simulink model "NavFilterTestHarness24"  (R2024b)
settings: Solver=FixedStepDiscrete  StartTime=startTime  StopTime=endTime  FixedStep=0.001  RelTol=1e-3  EnableMultiTasking=on
undefined symbols (not defined in the file): accel, ADSframe, ADStime, alignTime, angRate, ATTframe, CourseDeg, EAS2TAS, GndSpd, GPSframe, GPStime, Hgt, IMUframe, IMUtime, LatDeg, LngDeg, MagBiasX, MagBiasY, MagBiasZ, MAGframe, MAGtime, MagX, MagY, MagZ, msecHgtDelay, msecMagDelay, msecPosDelay, msecTasDelay, msecVelDelay, Pitch, Roll, Veas, VelD, Yaw
libraries: simulink x9, simulink_need_slupdate x2
(part 3 of 5)

== matlab function NavFilterTestHarness24/WatchDog/wrapAnglePi ==
  data: angleOut output; angleIn input
function angleOut   = wrapAnglePi(angleIn)
%#codegen

if abs(angleIn) <= pi
    angleOut = angleIn;
elseif  angleIn < -pi
    angleOut = angleIn + 2*pi;
elseif angleIn > pi
    angleOut = angleIn - 2*pi;
else
    angleOut = angleIn;
end

end

== matlab function NavFilterTestHarness24/InertialNavFilter/Predict States ==
  data: nextStates output; correctedDelAng output; correctedDelVel output; accNavMag output; states input; earthRateNED input; dAngIMU input; dVelIMU input; dtIMU input
%#codegen
function [nextStates,correctedDelAng,correctedDelVel,accNavMag]  = UpdateStrapdownEquationsNED( ...
    states, ...
    earthRateNED, ...
    dAngIMU, ...
    dVelIMU, ...
    dtIMU)

% define persistent variables for previous delta angle and velocity which
% are required for sculling and coning error corrections
persistent prevDelAng;
if isempty(prevDelAng)
    prevDelAng = single([0;0;0]);
end
persistent Tbn;
if isempty(Tbn)
    Tbn = single(eye(3));
end

gravityNED = [0.0;0.0;9.80665];

% Remove sensor bias errors
correctedDelAng = dAngIMU - states(11:13);
correctedDelVel = dVelIMU - states(14:16);

% Save current measurements
prevDelAng = correctedDelAng;

% Apply corrections for earths rotation rate and coning errors
correctedDelAng   = correctedDelAng - transpose(Tbn)*earthRateNED*dtIMU + 8.333333333333333e-2*cross(prevDelAng , dAngIMU);

% Initialise the updated state vector
nextStates   = states;

% Convert the rotation vector to its equivalent quaternion
rotationMag = sqrt(correctedDelAng(1)^2 + correctedDelAng(2)^2 + correctedDelAng(3)^2);
if rotationMag<1e-12
  deltaQuat = single([1;0;0;0]);
else
  deltaQuat = [cos(0.5*rotationMag); correctedDelAng/rotationMag*sin(0.5*rotationMag)];
end

% Update the quaternions by rotating from the previous attitude through
% the delta angle rotation quaternion
qUpdated = [states(1)*deltaQuat(1)-transpose(states(2:4))*deltaQuat(2:4); states(1)*deltaQuat(2:4) + deltaQuat(1)*states(2:4) + cross(states(2:4),deltaQuat(2:4))];

% Normalise the quaternions and update the quaternion states
quatMag = sqrt(qUpdated(1)^2 + qUpdated(2)^2 + qUpdated(3)^2 + qUpdated(4)^2);
if (quatMag < 1e-16)
    nextStates(1:4) = qUpdated;
else
    nextStates(1:4) = qUpdated / quatMag;
end

% Calculate the body to nav cosine matrix
Tbn = [nextStates(1)^2 + nextStates(2)^2 - nextStates(3)^2 - nextStates(4)^2, 2*(nextStates(2)*nextStates(3) - nextStates(1)*nextStates(4)), 2*(nextStates(2)*nextStates(4) + nextStates(1)*nextStates(3));...
      2*(nextStates(2)*nextStates(3) + nextStates(1)*nextStates(4)), nextStates(1)^2 - nextStates(2)^2 + nextStates(3)^2 - nextStates(4)^2, 2*(nextStates(3)*nextStates(4) - nextStates(1)*nextStates(2));...
      2*(nextStates(2)*nextStates(4)-nextStates(1)*nextStates(3)), 2*(nextStates(3)*nextStates(4) + nextStates(1)*nextStates(2)), nextStates(1)^2 - nextStates(2)^2 - nextStates(3)^2 + nextStates(4)^2];
  
% transform body delta velocities to delta velocities in the nav frame
delVelNav = Tbn * correctedDelVel + gravityNED*dtIMU;

% calculate the magnitude of the nav acceleration (required for GPS
% variance estimation)
accNavMag = sqrt(delVelNav(1)^2 + delVelNav(2)^2 + delVelNav(3)^2) / dtIMU;

% If calculating position save previous velocity
lastVelocity = nextStates(5:7);

% Sum delta velocities to get velocity after removing gravitational skew and correcting for transport rate
nextStates(5:7) = states(5:7) + delVelNav;


% If calculating postions, do a trapezoidal integration for position
nextStates(8:10)     = states(8:10) + 0.5*(nextStates(5:7) + lastVelocity)*dtIMU;

% Copy the remaining states across
nextStates(11:24) = states(11:24);

end
